simulink model "Week11_Simulation_Control"  (R2017b)
settings: Solver=ode4  StartTime=0.0  StopTime=20  FixedStep=1e-3  RelTol=1e-3  EnableMultiTasking=on
values from neighbouring files (symbols this model uses):
  g = 9.8    [Parameters.m]
  l1 = 3    [Parameters.m]
  l2 = 2    [Parameters.m]
  m1 = 3    [Parameters.m]
  m2 = 2    [Parameters.m]
undefined symbols (not defined in the file or in its folder): DiscIntNeverNeededParam
libraries: simulink x16, dspinverses x6
(part 1 of 2)
settings Model: Creator=e27269  LastModifiedBy=e27269
settings DataIOCC: LimitDataPoints=on
settings OptimizationCC: LifeSpan=inf
settings DebuggingCC: AllowSymbolicDim=off  SFUnexpectedBacktrackingDiag=warning  SFNoUnconditionalDefaultTransitionDiag=warning  SFExecutionAtInitializationDiag=none
settings ModelReferenceCC: PropagateSignalLabelsOutOfModel=off
settings CodeAppCC: StateflowObjectComments=on
settings GRTTargetCC: TargetLangStandard=C89/C90 (ANSI)
settings ConfigComp: CovMetricSettings=dw  CovHtmlReporting=on  CovSaveCumulativeToWorkspaceVar=on  CovSaveSingleToWorkspaceVar=on  CovExternalEMLEnable=off

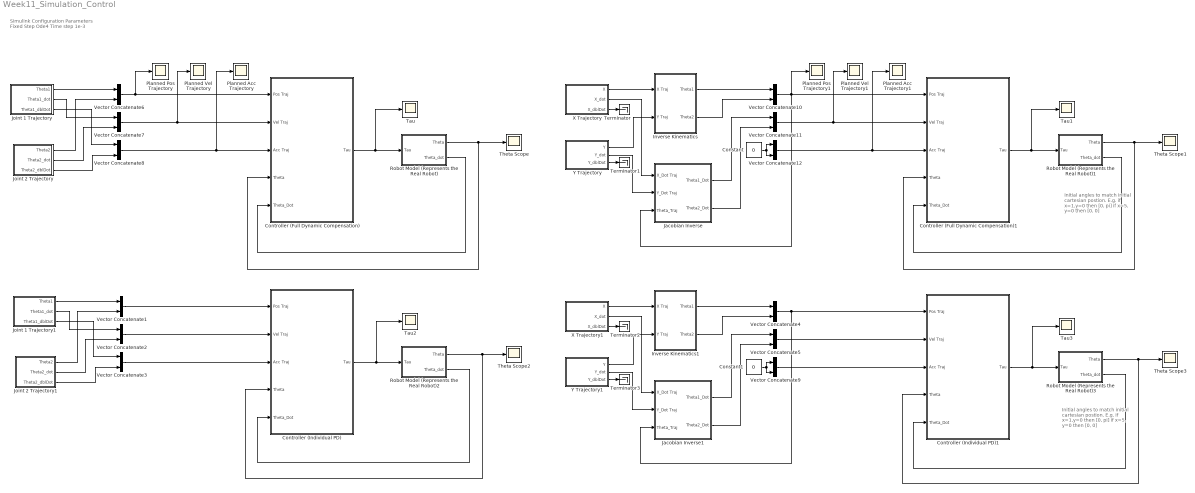
== system Week11_Simulation_Control ==
  note: Simulink Configuration Parameters
      | Fixed Step
      | Ode4
      | Time step 1e-3
  note: Initial angles to
      | match initial
      | cartesian postion.
      | E.g. if x=1,y=0
      | then [0, pi]
      | if x=5, y=0
      | then [0, 0]
  note: Initial angles to
      | match initial
      | cartesian postion.
      | E.g. if x=1,y=0
      | then [0, pi]
      | if x=5, y=0
      | then [0, 0]
  Constant : Constant  Value=0
  Constant1 : Constant  Value=0
  Controller (Full Dynamic Compensation) : Subsystem
  Controller (Full Dynamic Compensation)1 : Subsystem
  Controller (Individual PD) : Subsystem
  Controller (Individual PD)1 : Subsystem
  Inverse Kinematics : Subsystem
  Inverse Kinematics1 : Subsystem
  Jacobian Inverse : Subsystem
  Jacobian Inverse1 : Subsystem
  Joint 1 Trajectory : Subsystem
  Joint 1 Trajectory1 : Subsystem
  Joint 2 Trajectory : Subsystem
  Joint 2 Trajectory1 : Subsystem
  Planned Acc Trajectory : Scope
  Planned Acc Trajectory1 : Scope
  Planned Pos Trajectory : Scope
  Planned Pos Trajectory1 : Scope
  Planned Vel Trajectory : Scope
  Planned Vel Trajectory1 : Scope
  Robot Model (Represents the Real Robot) : Subsystem
  Robot Model (Represents the Real Robot)1 : Subsystem
  Robot Model (Represents the Real Robot)2 : Subsystem
  Robot Model (Represents the Real Robot)3 : Subsystem
  Tau{,1..3} (4 alike) : Scope
  Terminator{,1..3} (4 alike) : Terminator
  Theta Scope{,1..3} (4 alike) : Scope
  Vector Concatenate{1..12} (12 alike) : Concatenate  Mode=Multidimensional array
  X Trajectory : Subsystem
  X Trajectory1 : Subsystem
  Y Trajectory : Subsystem
  Y Trajectory1 : Subsystem
  wires:
  Joint 1 Trajectory/1(Theta1) -> Vector Concatenate6/1
  Joint 2 Trajectory/2(Theta2_dot) -> Vector Concatenate7/2
  Joint 2 Trajectory/1(Theta2) -> Vector Concatenate6/2
  Joint 1 Trajectory/2(Theta1_dot) -> Vector Concatenate7/1
  Joint 1 Trajectory/3(Theta1_dblDot) -> Vector Concatenate8/1
  Joint 2 Trajectory/3(Theta2_dblDot) -> Vector Concatenate8/2
  Vector Concatenate6/1 -> Controller (Full Dynamic Compensation)/1(Pos Traj), Planned Pos Trajectory/1
  Vector Concatenate7/1 -> Planned Vel Trajectory/1, Controller (Full Dynamic Compensation)/2(Vel Traj)
  Robot Model (Represents the Real Robot)/1(Theta) -> Controller (Full Dynamic Compensation)/4(Theta), Theta Scope/1
  Vector Concatenate8/1 -> Planned Acc Trajectory/1, Controller (Full Dynamic Compensation)/3(Acc Traj)
  Controller (Full Dynamic Compensation)/1(Tau) -> Tau/1, Robot Model (Represents the Real Robot)/1(Tau)
  Robot Model (Represents the Real Robot)/2(Theta_dot) -> Controller (Full Dynamic Compensation)/5(Theta_Dot)
  Robot Model (Represents the Real Robot)2/2(Theta_dot) -> Controller (Individual PD)/5(Theta_Dot)
  Controller (Individual PD)/1(Tau) -> Robot Model (Represents the Real Robot)2/1(Tau), Tau2/1
  Robot Model (Represents the Real Robot)2/1(Theta) -> Controller (Individual PD)/4(Theta), Theta Scope2/1
  Joint 2 Trajectory1/3(Theta2_dblDot) -> Vector Concatenate3/2
  Joint 2 Trajectory1/1(Theta2) -> Vector Concatenate1/2
  Joint 1 Trajectory1/3(Theta1_dblDot) -> Vector Concatenate3/1
  Joint 1 Trajectory1/2(Theta1_dot) -> Vector Concatenate2/1
  Joint 2 Trajectory1/2(Theta2_dot) -> Vector Concatenate2/2
  Joint 1 Trajectory1/1(Theta1) -> Vector Concatenate1/1
  Vector Concatenate1/1 -> Controller (Individual PD)/1(Pos Traj)
  Vector Concatenate2/1 -> Controller (Individual PD)/2(Vel Traj)
  Vector Concatenate3/1 -> Controller (Individual PD)/3(Acc Traj)
  Jacobian Inverse1/1(Theta1_Dot) -> Vector Concatenate5/1
  Y Trajectory1/1(Y) -> Inverse Kinematics1/2(Y Traj)
  Inverse Kinematics1/1(Theta1) -> Vector Concatenate4/1
  Vector Concatenate4/1 -> Controller (Individual PD)1/1(Pos Traj), Jacobian Inverse1/3(Theta_Traj)
  Vector Concatenate5/1 -> Controller (Individual PD)1/2(Vel Traj)
  Jacobian Inverse1/2(Theta2_Dot) -> Vector Concatenate5/2
  X Trajectory1/2(X_dot) -> Jacobian Inverse1/1(X_Dot Traj)
  X Trajectory/2(X_dot) -> Jacobian Inverse/1(X_Dot Traj)
  Jacobian Inverse/2(Theta2_Dot) -> Vector Concatenate11/2
  Robot Model (Represents the Real Robot)3/2(Theta_dot) -> Controller (Individual PD)1/5(Theta_Dot)
  Constant/1 -> Vector Concatenate12/2, Vector Concatenate12/1
  Vector Concatenate11/1 -> Planned Vel Trajectory1/1, Controller (Full Dynamic Compensation)1/2(Vel Traj)
  Robot Model (Represents the Real Robot)1/1(Theta) -> Controller (Full Dynamic Compensation)1/4(Theta), Theta Scope1/1
  Vector Concatenate10/1 -> Jacobian Inverse/3(Theta_Traj), Controller (Full Dynamic Compensation)1/1(Pos Traj), Planned Pos Trajectory1/1
  X Trajectory/1(X) -> Inverse Kinematics/1(X Traj)
  Y Trajectory1/3(Y_dblDot) -> Terminator3/1
  Controller (Individual PD)1/1(Tau) -> Robot Model (Represents the Real Robot)3/1(Tau), Tau3/1
  Inverse Kinematics/1(Theta1) -> Vector Concatenate10/1
  Robot Model (Represents the Real Robot)3/1(Theta) -> Controller (Individual PD)1/4(Theta), Theta Scope3/1
  Y Trajectory/1(Y) -> Inverse Kinematics/2(Y Traj)
  Jacobian Inverse/1(Theta1_Dot) -> Vector Concatenate11/1
  Robot Model (Represents the Real Robot)1/2(Theta_dot) -> Controller (Full Dynamic Compensation)1/5(Theta_Dot)
  X Trajectory1/1(X) -> Inverse Kinematics1/1(X Traj)
  Controller (Full Dynamic Compensation)1/1(Tau) -> Tau1/1, Robot Model (Represents the Real Robot)1/1(Tau)
  Vector Concatenate12/1 -> Planned Acc Trajectory1/1, Controller (Full Dynamic Compensation)1/3(Acc Traj)
  Inverse Kinematics/2(Theta2) -> Vector Concatenate10/2
  X Trajectory/3(X_dblDot) -> Terminator/1
  Y Trajectory1/2(Y_dot) -> Jacobian Inverse1/2(Y_Dot Traj)
  Inverse Kinematics1/2(Theta2) -> Vector Concatenate4/2
  Vector Concatenate9/1 -> Controller (Individual PD)1/3(Acc Traj)
  Y Trajectory/3(Y_dblDot) -> Terminator1/1
  X Trajectory1/3(X_dblDot) -> Terminator2/1
  Y Trajectory/2(Y_dot) -> Jacobian Inverse/2(Y_Dot Traj)
  Constant1/1 -> Vector Concatenate9/2, Vector Concatenate9/1

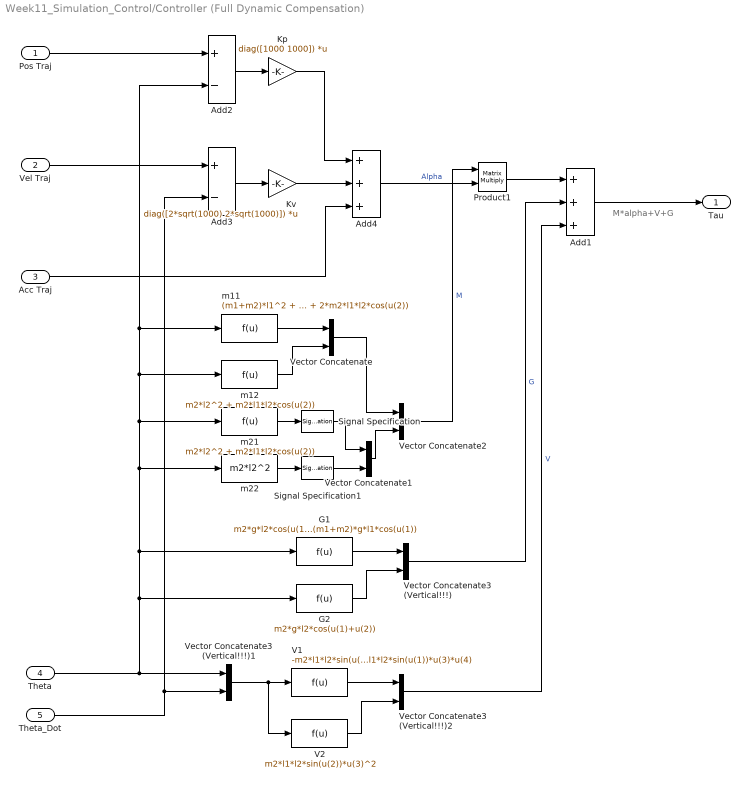
== system Week11_Simulation_Control/Controller (Full Dynamic Compensation) ==
  note: M*alpha+V+G
  Pos Traj : Inport
  Vel Traj : Inport  Port=2
  Acc Traj : Inport  Port=3
  Theta : Inport  Port=4
  Theta_Dot : Inport  Port=5
  Add1 : Sum  Inputs=+++
  Add2 : Sum  Inputs=+-
  Add3 : Sum  Inputs=+-
  Add4 : Sum  Inputs=+++
  G1 : Fcn  Expr=m2*g*l2*cos(u(1)+u(2))+(m1+m2)*g*l1*cos(u(1))
  G2 : Fcn  Expr=m2*g*l2*cos(u(1)+u(2))
  Kp : Gain  Gain=diag([1000 1000])  Multiplication=Matrix(K*u) (u vector)
  Kv : Gain  Gain=diag([2*sqrt(1000) 2*sqrt(1000)])  Multiplication=Matrix(K*u) (u vector)
  Product1 : Product  Multiplication=Matrix(*)
  Signal Specification : SignalSpecification  Dimensions=[1,1]
  Signal Specification1 : SignalSpecification  Dimensions=[1,1]
  V1 : Fcn  Expr=-m2*l1*l2*sin(u(2))*u(4)^2-2*m2*l1*l2*sin(u(1))*u(3)*u(4)
  V2 : Fcn  Expr=m2*l1*l2*sin(u(2))*u(3)^2
  Vector Concatenate : Concatenate  Mode=Multidimensional array  ConcatenateDimension=2
  Vector Concatenate1 : Concatenate  Mode=Multidimensional array  ConcatenateDimension=2
  Vector Concatenate2 : Concatenate  Mode=Multidimensional array
  Vector Concatenate3 (Vertical!!!) : Concatenate  Mode=Multidimensional array
  Vector Concatenate3 (Vertical!!!)1 : Concatenate  Mode=Multidimensional array
  Vector Concatenate3 (Vertical!!!)2 : Concatenate  Mode=Multidimensional array
  m11 : Fcn  Expr=(m1+m2)*l1^2 + m2*l2^2 + 2*m2*l1*l2*cos(u(2))
  m12 : Fcn  Expr=m2*l2^2 + m2*l1*l2*cos(u(2))
  m21 : Fcn  Expr=m2*l2^2 + m2*l1*l2*cos(u(2))
  m22 : Fcn  Expr=m2*l2^2
  Tau : Outport
  wires:
  Vector Concatenate3 (Vertical!!!)2/1 -> Add1/3  "V"
  Vector Concatenate3 (Vertical!!!)1/1 -> V2/1, V1/1
  Theta_Dot/1 -> Vector Concatenate3 (Vertical!!!)1/2, Add3/2
  V1/1 -> Vector Concatenate3 (Vertical!!!)2/1
  Pos Traj/1 -> Add2/1
  Theta/1 -> Add2/2, m11/1, m12/1, m21/1, m22/1, G1/1, G2/1, Vector Concatenate3 (Vertical!!!)1/1
  Signal Specification/1 -> Vector Concatenate1/1
  Vel Traj/1 -> Add3/1
  V2/1 -> Vector Concatenate3 (Vertical!!!)2/2
  Vector Concatenate1/1 -> Vector Concatenate2/2
  Vector Concatenate/1 -> Vector Concatenate2/1
  Signal Specification1/1 -> Vector Concatenate1/2
  m12/1 -> Vector Concatenate/2
  G2/1 -> Vector Concatenate3 (Vertical!!!)/2
  G1/1 -> Vector Concatenate3 (Vertical!!!)/1
  Vector Concatenate2/1 -> Product1/1  "M"
  Acc Traj/1 -> Add4/3
  m22/1 -> Signal Specification1/1
  m11/1 -> Vector Concatenate/1
  m21/1 -> Signal Specification/1
  Add1/1 -> Tau/1
  Vector Concatenate3 (Vertical!!!)/1 -> Add1/2  "G"
  Product1/1 -> Add1/1
  Add2/1 -> Kp/1
  Add3/1 -> Kv/1
  Kv/1 -> Add4/2
  Kp/1 -> Add4/1
  Add4/1 -> Product1/2  "Alpha"

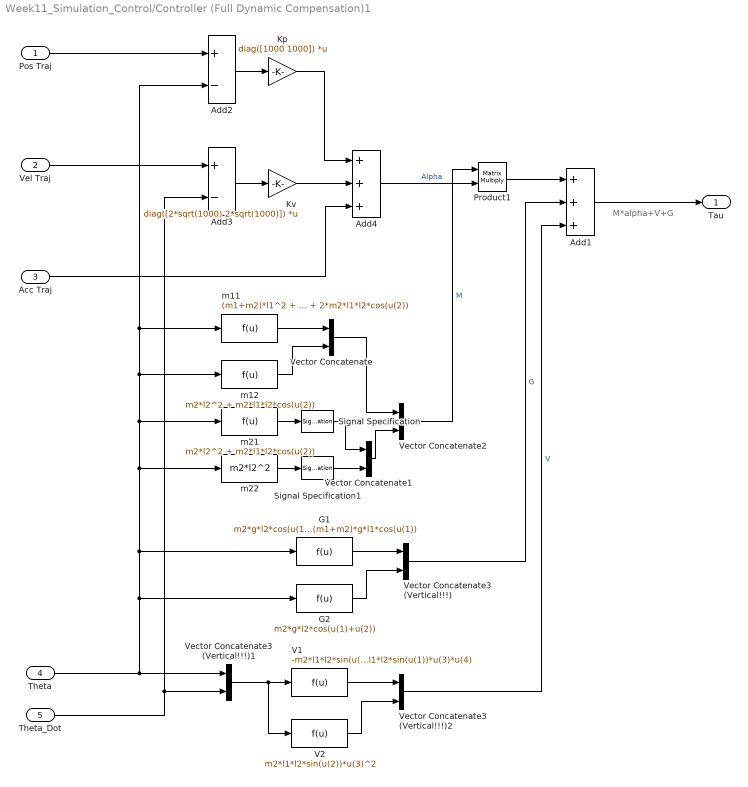
== system Week11_Simulation_Control/Controller (Full Dynamic Compensation)1 ==
  note: M*alpha+V+G
  Pos Traj : Inport
  Vel Traj : Inport  Port=2
  Acc Traj : Inport  Port=3
  Theta : Inport  Port=4
  Theta_Dot : Inport  Port=5
  Add1 : Sum  Inputs=+++
  Add2 : Sum  Inputs=+-
  Add3 : Sum  Inputs=+-
  Add4 : Sum  Inputs=+++
  G1 : Fcn  Expr=m2*g*l2*cos(u(1)+u(2))+(m1+m2)*g*l1*cos(u(1))
  G2 : Fcn  Expr=m2*g*l2*cos(u(1)+u(2))
  Kp : Gain  Gain=diag([1000 1000])  Multiplication=Matrix(K*u) (u vector)
  Kv : Gain  Gain=diag([2*sqrt(1000) 2*sqrt(1000)])  Multiplication=Matrix(K*u) (u vector)
  Product1 : Product  Multiplication=Matrix(*)
  Signal Specification : SignalSpecification  Dimensions=[1,1]
  Signal Specification1 : SignalSpecification  Dimensions=[1,1]
  V1 : Fcn  Expr=-m2*l1*l2*sin(u(2))*u(4)^2-2*m2*l1*l2*sin(u(1))*u(3)*u(4)
  V2 : Fcn  Expr=m2*l1*l2*sin(u(2))*u(3)^2
  Vector Concatenate : Concatenate  Mode=Multidimensional array  ConcatenateDimension=2
  Vector Concatenate1 : Concatenate  Mode=Multidimensional array  ConcatenateDimension=2
  Vector Concatenate2 : Concatenate  Mode=Multidimensional array
  Vector Concatenate3 (Vertical!!!) : Concatenate  Mode=Multidimensional array
  Vector Concatenate3 (Vertical!!!)1 : Concatenate  Mode=Multidimensional array
  Vector Concatenate3 (Vertical!!!)2 : Concatenate  Mode=Multidimensional array
  m11 : Fcn  Expr=(m1+m2)*l1^2 + m2*l2^2 + 2*m2*l1*l2*cos(u(2))
  m12 : Fcn  Expr=m2*l2^2 + m2*l1*l2*cos(u(2))
  m21 : Fcn  Expr=m2*l2^2 + m2*l1*l2*cos(u(2))
  m22 : Fcn  Expr=m2*l2^2
  Tau : Outport
  wires:
  Vector Concatenate3 (Vertical!!!)2/1 -> Add1/3  "V"
  Vector Concatenate3 (Vertical!!!)1/1 -> V2/1, V1/1
  Theta_Dot/1 -> Vector Concatenate3 (Vertical!!!)1/2, Add3/2
  V1/1 -> Vector Concatenate3 (Vertical!!!)2/1
  Pos Traj/1 -> Add2/1
  Theta/1 -> Add2/2, m11/1, m12/1, m21/1, m22/1, G1/1, G2/1, Vector Concatenate3 (Vertical!!!)1/1
  Signal Specification/1 -> Vector Concatenate1/1
  Vel Traj/1 -> Add3/1
  V2/1 -> Vector Concatenate3 (Vertical!!!)2/2
  Vector Concatenate1/1 -> Vector Concatenate2/2
  Vector Concatenate/1 -> Vector Concatenate2/1
  Signal Specification1/1 -> Vector Concatenate1/2
  m12/1 -> Vector Concatenate/2
  G2/1 -> Vector Concatenate3 (Vertical!!!)/2
  G1/1 -> Vector Concatenate3 (Vertical!!!)/1
  Vector Concatenate2/1 -> Product1/1  "M"
  Acc Traj/1 -> Add4/3
  m22/1 -> Signal Specification1/1
  m11/1 -> Vector Concatenate/1
  m21/1 -> Signal Specification/1
  Add1/1 -> Tau/1
  Vector Concatenate3 (Vertical!!!)/1 -> Add1/2  "G"
  Product1/1 -> Add1/1
  Add2/1 -> Kp/1
  Add3/1 -> Kv/1
  Kv/1 -> Add4/2
  Kp/1 -> Add4/1
  Add4/1 -> Product1/2  "Alpha"

== system Week11_Simulation_Control/Controller (Individual PD) ==
  Pos Traj : Inport
  Vel Traj : Inport  Port=2
  Acc Traj : Inport  Port=3
  Theta : Inport  Port=4
  Theta_Dot : Inport  Port=5
  Add2 : Sum  Inputs=+-
  Add3 : Sum  Inputs=+-
  Add4 : Sum  Inputs=+++
  Kp : Gain  Gain=diag([4000 4000])  Multiplication=Matrix(K*u) (u vector)
  Kv : Gain  Gain=diag([2*sqrt(4000) 2*sqrt(4000)])  Multiplication=Matrix(K*u) (u vector)
  Tau : Outport
  wires:
  Theta_Dot/1 -> Add3/2
  Pos Traj/1 -> Add2/1
  Theta/1 -> Add2/2
  Vel Traj/1 -> Add3/1
  Acc Traj/1 -> Add4/3
  Add2/1 -> Kp/1
  Add3/1 -> Kv/1
  Kv/1 -> Add4/2
  Kp/1 -> Add4/1
  Add4/1 -> Tau/1  "PD Control"

== system Week11_Simulation_Control/Controller (Individual PD)1 ==
  Pos Traj : Inport
  Vel Traj : Inport  Port=2
  Acc Traj : Inport  Port=3
  Theta : Inport  Port=4
  Theta_Dot : Inport  Port=5
  Add2 : Sum  Inputs=+-
  Add3 : Sum  Inputs=+-
  Add4 : Sum  Inputs=+++
  Kp : Gain  Gain=diag([4000 4000])  Multiplication=Matrix(K*u) (u vector)
  Kv : Gain  Gain=diag([2*sqrt(4000) 2*sqrt(4000)])  Multiplication=Matrix(K*u) (u vector)
  Tau : Outport
  wires:
  Theta_Dot/1 -> Add3/2
  Pos Traj/1 -> Add2/1
  Theta/1 -> Add2/2
  Vel Traj/1 -> Add3/1
  Acc Traj/1 -> Add4/3
  Add2/1 -> Kp/1
  Add3/1 -> Kv/1
  Kv/1 -> Add4/2
  Kp/1 -> Add4/1
  Add4/1 -> Tau/1  "PD Control"

== system Week11_Simulation_Control/Inverse Kinematics ==
  X Traj : Inport
  Y Traj : Inport  Port=2
  Add : Sum  Inputs=++--
  Add2 : Sum  Inputs=+++-
  Add3 : Sum
  Add4 : Sum  Inputs=+-
  Constant : Constant  Value=l1^2
  Constant1 : Constant  Value=l2^2
  Constant2 : Constant  Value=2*l1*l2
  Constant3 : Constant  Value=l1^2
  Constant4 : Constant  Value=l2^2
  Constant5 : Constant  Value=2*l1
  Divide : Product  Inputs=*/
  Divide1 : Product  Inputs=*//
  Product : Product
  Product1 : Product
  Sqrt : Sqrt  SaturateOnIntegerOverflow=on
  Trigonometric Function : Trigonometry  Operator=acos
  Trigonometric Function1 : Trigonometry  Operator=atan2
  Trigonometric Function2 : Trigonometry  Operator=acos
  Theta1 : Outport
  Theta2 : Outport  Port=2
  wires:
  X Traj/1 -> Trigonometric Function1/2, Product/2, Product/1  "x"
  Y Traj/1 -> Trigonometric Function1/1, Product1/2, Product1/1  "y"
  Product/1 -> Add3/1, Add2/2, Add/1
  Constant/1 -> Add/3
  Constant1/1 -> Add/4
  Add/1 -> Divide/1
  Constant2/1 -> Divide/2
  Divide/1 -> Trigonometric Function/1
  Trigonometric Function/1 -> Theta2/1
  Trigonometric Function1/1 -> Add4/1  "beta"
  Constant3/1 -> Add2/1
  Constant4/1 -> Add2/4
  Add2/1 -> Divide1/1
  Constant5/1 -> Divide1/2
  Product1/1 -> Add3/2, Add2/3, Add/2
  Add3/1 -> Sqrt/1
  Sqrt/1 -> Divide1/3
  Divide1/1 -> Trigonometric Function2/1
  Trigonometric Function2/1 -> Add4/2  "psi"
  Add4/1 -> Theta1/1

== system Week11_Simulation_Control/Inverse Kinematics1 ==
  X Traj : Inport
  Y Traj : Inport  Port=2
  Add : Sum  Inputs=++--
  Add2 : Sum  Inputs=+++-
  Add3 : Sum
  Add4 : Sum  Inputs=+-
  Constant : Constant  Value=l1^2
  Constant1 : Constant  Value=l2^2
  Constant2 : Constant  Value=2*l1*l2
  Constant3 : Constant  Value=l1^2
  Constant4 : Constant  Value=l2^2
  Constant5 : Constant  Value=2*l1
  Divide : Product  Inputs=*/
  Divide1 : Product  Inputs=*//
  Product : Product
  Product1 : Product
  Sqrt : Sqrt  SaturateOnIntegerOverflow=on
  Trigonometric Function : Trigonometry  Operator=acos
  Trigonometric Function1 : Trigonometry  Operator=atan2
  Trigonometric Function2 : Trigonometry  Operator=acos
  Theta1 : Outport
  Theta2 : Outport  Port=2
  wires:
  X Traj/1 -> Trigonometric Function1/2, Product/2, Product/1  "x"
  Y Traj/1 -> Trigonometric Function1/1, Product1/2, Product1/1  "y"
  Product/1 -> Add3/1, Add2/2, Add/1
  Constant/1 -> Add/3
  Constant1/1 -> Add/4
  Add/1 -> Divide/1
  Constant2/1 -> Divide/2
  Divide/1 -> Trigonometric Function/1
  Trigonometric Function/1 -> Theta2/1
  Trigonometric Function1/1 -> Add4/1  "beta"
  Constant3/1 -> Add2/1
  Constant4/1 -> Add2/4
  Add2/1 -> Divide1/1
  Constant5/1 -> Divide1/2
  Product1/1 -> Add3/2, Add2/3, Add/2
  Add3/1 -> Sqrt/1
  Sqrt/1 -> Divide1/3
  Divide1/1 -> Trigonometric Function2/1
  Trigonometric Function2/1 -> Add4/2  "psi"
  Add4/1 -> Theta1/1

== system Week11_Simulation_Control/Jacobian Inverse ==
  note: vertical
  note: vertical
  note: horizontal
  note: horizontal
  X_Dot Traj : Inport
  Y_Dot Traj : Inport  Port=2
  Theta_Traj : Inport  Port=3
  Demux : Demux  Outputs=2
  J11 : Fcn  Expr=-l1*sin(u(1))-l2*sin(u(1)+u(2))
  J12 : Fcn  Expr=-l2*sin(u(1)+u(2))
  J21 : Fcn  Expr=l1*cos(u(1))+l2*cos(u(1)+u(2))
  J22 : Fcn  Expr=l2*cos(u(1)+u(2))
  Product : Product  Multiplication=Matrix(*)
  Pseudoinverse : dspinverses/Pseudoinverse  wanterr=off  SimulateUsing=Interpreted execution
      settings: SourceProductName=DSP System Toolbox  SourceProductBaseCode=DS
  Vector Concatenate : Concatenate  Mode=Multidimensional array  ConcatenateDimension=2
  Vector Concatenate1 : Concatenate  Mode=Multidimensional array  ConcatenateDimension=2
  Vector Concatenate2 : Concatenate  Mode=Multidimensional array
  Vector Concatenate3 : Concatenate  Mode=Multidimensional array
  Theta1_Dot : Outport
  Theta2_Dot : Outport  Port=2
  wires:
  Theta_Traj/1 -> J21/1, J22/1, J12/1, J11/1
  J11/1 -> Vector Concatenate/1
  J12/1 -> Vector Concatenate/2
  J21/1 -> Vector Concatenate1/1
  J22/1 -> Vector Concatenate1/2
  Vector Concatenate/1 -> Vector Concatenate2/1
  Vector Concatenate1/1 -> Vector Concatenate2/2
  Vector Concatenate2/1 -> Pseudoinverse/1  "J"
  X_Dot Traj/1 -> Vector Concatenate3/1  "x_dot"
  Y_Dot Traj/1 -> Vector Concatenate3/2  "y_dot"
  Pseudoinverse/1 -> Product/1  "Jinv"
  Vector Concatenate3/1 -> Product/2  "v"
  Product/1 -> Demux/1
  Demux/1 -> Theta1_Dot/1
  Demux/2 -> Theta2_Dot/1

== system Week11_Simulation_Control/Jacobian Inverse1 ==
  note: vertical
  note: vertical
  note: horizontal
  note: horizontal
  X_Dot Traj : Inport
  Y_Dot Traj : Inport  Port=2
  Theta_Traj : Inport  Port=3
  Demux : Demux  Outputs=2
  J11 : Fcn  Expr=-l1*sin(u(1))-l2*sin(u(1)+u(2))
  J12 : Fcn  Expr=-l2*sin(u(1)+u(2))
  J21 : Fcn  Expr=l1*cos(u(1))+l2*cos(u(1)+u(2))
  J22 : Fcn  Expr=l2*cos(u(1)+u(2))
  Product : Product  Multiplication=Matrix(*)
  Pseudoinverse : dspinverses/Pseudoinverse  wanterr=off  SimulateUsing=Interpreted execution
      settings: SourceProductName=DSP System Toolbox  SourceProductBaseCode=DS
  Vector Concatenate : Concatenate  Mode=Multidimensional array  ConcatenateDimension=2
  Vector Concatenate1 : Concatenate  Mode=Multidimensional array  ConcatenateDimension=2
  Vector Concatenate2 : Concatenate  Mode=Multidimensional array
  Vector Concatenate3 : Concatenate  Mode=Multidimensional array
  Theta1_Dot : Outport
  Theta2_Dot : Outport  Port=2
  wires:
  Theta_Traj/1 -> J21/1, J22/1, J12/1, J11/1
  J11/1 -> Vector Concatenate/1
  J12/1 -> Vector Concatenate/2
  J21/1 -> Vector Concatenate1/1
  J22/1 -> Vector Concatenate1/2
  Vector Concatenate/1 -> Vector Concatenate2/1
  Vector Concatenate1/1 -> Vector Concatenate2/2
  Vector Concatenate2/1 -> Pseudoinverse/1  "J"
  X_Dot Traj/1 -> Vector Concatenate3/1  "x_dot"
  Y_Dot Traj/1 -> Vector Concatenate3/2  "y_dot"
  Pseudoinverse/1 -> Product/1  "Jinv"
  Vector Concatenate3/1 -> Product/2  "v"
  Product/1 -> Demux/1
  Demux/1 -> Theta1_Dot/1
  Demux/2 -> Theta2_Dot/1

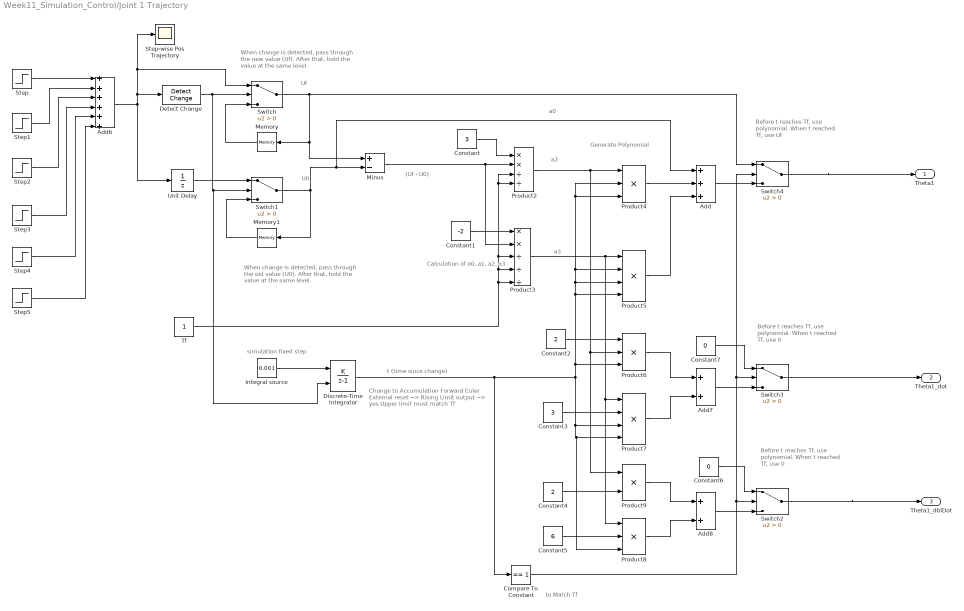
== system Week11_Simulation_Control/Joint 1 Trajectory ==
  note: Generate Polynomial
  note: Calculation of
      | a0, a1, a2, a3
  note: Before t reaches Tf,
      | use polynomial.
      | When t reached Tf,
      | use Uf
  note: to Match Tf
  note: t (time since change)
  note: When change is detected, pass through
      | the old value (U0). After that, hold the
      | value at the same level.
  note: simulation fixed step
  note: Change to Accumulation Forward Euler
      | External reset --> Rising
      | Limit output --> yes
      | Upper limit must match Tf
  note: a3
  note: a2
  note: Uf
  note: U0
  note: When change is detected, pass through
      | the new value (Uf). After that, hold the
      | value at the same level.
  note: Before t reaches Tf,
      | use polynomial.
      | When t reached Tf,
      | use 0
  note: Before t reaches Tf,
      | use polynomial.
      | When t reached Tf,
      | use 0
  note: (Uf - U0)
  note: a0
  Add : Sum  Inputs=3
  Add6 : Sum  Inputs=6
  Add7 : Sum  Inputs=2
  Add8 : Sum  Inputs=2
  Compare To Constant : simulink/Logic and Bit Operations/Compare To Constant  relop===  const=1  OutDataTypeStr=boolean
  Constant : Constant  Value=3
  Constant1 : Constant  Value=-2
  Constant2 : Constant  Value=2
  Constant3 : Constant  Value=3
  Constant4 : Constant  Value=2
  Constant5 : Constant  Value=6
  Constant6 : Constant  Value=0
  Constant7 : Constant  Value=0
  Detect Change : simulink/Logic and Bit Operations/Detect Change  vinit=0  InputProcessing=Inherited  OutDataTypeStr=boolean
  Discrete-Time Integrator : DiscreteIntegrator  IntegratorMethod=Accumulation: Forward Euler  gainval=1  ExternalReset=rising  InitialConditionSetting=State (most efficient)  SampleTime=-1  LimitOutput=on  UpperSaturationLimit=1  ICPrevOutput=DiscIntNeverNeededParam  ICPrevScaledInput=DiscIntNeverNeededParam
  Integral source : Constant  Value=0.001
  Memory : Memory  InheritSampleTime=on
  Memory1 : Memory  InheritSampleTime=on
  Minus : Sum  Inputs=+-
  Product2 : Product  Inputs=**//
  Product3 : Product  Inputs=**///
  Product4 : Product  Inputs=3
  Product5 : Product  Inputs=4
  Product6 : Product  Inputs=3
  Product7 : Product  Inputs=4
  Product8 : Product  Inputs=3
  Product9 : Product
  Step : Step  SampleTime=0
  Step-wise Pos Trajectory : Scope
  Step1 : Step  Time=4  After=2  SampleTime=0
  Step2 : Step  Time=8  After=-1  SampleTime=0
  Step3 : Step  Time=11  After=1.5  SampleTime=0
  Step4 : Step  Time=14  After=-1  SampleTime=0
  Step5 : Step  Time=17  After=-2  SampleTime=0
  Switch{,1..4} (5 alike) : Switch  Criteria=u2 > Threshold
  Tf : Constant
  Unit Delay : UnitDelay  SampleTime=-1
  Theta1 : Outport
  Theta1_dot : Outport  Port=2
  Theta1_dblDot : Outport  Port=3
  wires:
  Add8/1 -> Switch2/3
  Product9/1 -> Add8/1
  Constant7/1 -> Switch3/1
  Constant/1 -> Product2/1
  Step/1 -> Add6/1
  Integral source/1 -> Discrete-Time Integrator/1
  Switch4/1 -> Theta1/1
  Add/1 -> Switch4/3
  Add6/1 -> Switch/1, Step-wise Pos Trajectory/1, Detect Change/1, Unit Delay/1
  Product4/1 -> Add/2
  Switch3/1 -> Theta1_dot/1
  Compare To Constant/1 -> Switch4/2, Switch3/2, Switch2/2
  Switch2/1 -> Theta1_dblDot/1
  Step5/1 -> Add6/6
  Constant6/1 -> Switch2/1
  Step3/1 -> Add6/4
  Constant4/1 -> Product9/2
  Product8/1 -> Add8/2
  Constant5/1 -> Product8/2
  Product5/1 -> Add/3
  Product7/1 -> Add7/2
  Constant3/1 -> Product7/2
  Step4/1 -> Add6/5
  Detect Change/1 -> Discrete-Time Integrator/2, Switch1/2, Switch/2
  Step1/1 -> Add6/2
  Discrete-Time Integrator/1 -> Compare To Constant/1, Product7/3, Product8/3, Product7/4, Product6/3, Product5/4, Product5/3, Product5/2, Product4/3, Product4/2
  Product3/1 -> Product8/1, Product7/1, Product5/1
  Constant1/1 -> Product3/1
  Product6/1 -> Add7/1
  Tf/1 -> Product3/5, Product3/4, Product3/3, Product2/4, Product2/3
  Add7/1 -> Switch3/3
  Step2/1 -> Add6/3
  Minus/1 -> Product3/2, Product2/2
  Unit Delay/1 -> Switch1/1
  Memory1/1 -> Switch1/3
  Switch1/1 -> Memory1/1, Add/1, Minus/2
  Constant2/1 -> Product6/1
  Product2/1 -> Product9/1, Product6/2, Product4/1
  Memory/1 -> Switch/3
  Switch/1 -> Minus/1, Memory/1, Switch4/1

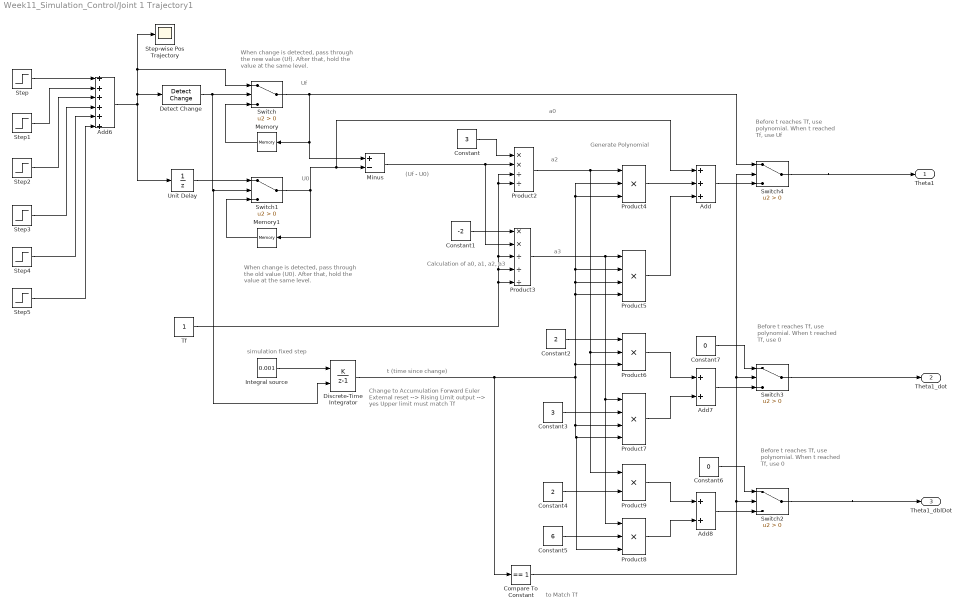
== system Week11_Simulation_Control/Joint 1 Trajectory1 ==
  note: Generate Polynomial
  note: Calculation of
      | a0, a1, a2, a3
  note: Before t reaches Tf,
      | use polynomial.
      | When t reached Tf,
      | use Uf
  note: to Match Tf
  note: t (time since change)
  note: When change is detected, pass through
      | the old value (U0). After that, hold the
      | value at the same level.
  note: simulation fixed step
  note: Change to Accumulation Forward Euler
      | External reset --> Rising
      | Limit output --> yes
      | Upper limit must match Tf
  note: a3
  note: a2
  note: Uf
  note: U0
  note: When change is detected, pass through
      | the new value (Uf). After that, hold the
      | value at the same level.
  note: Before t reaches Tf,
      | use polynomial.
      | When t reached Tf,
      | use 0
  note: Before t reaches Tf,
      | use polynomial.
      | When t reached Tf,
      | use 0
  note: (Uf - U0)
  note: a0
  Add : Sum  Inputs=3
  Add6 : Sum  Inputs=6
  Add7 : Sum  Inputs=2
  Add8 : Sum  Inputs=2
  Compare To Constant : simulink/Logic and Bit Operations/Compare To Constant  relop===  const=1  OutDataTypeStr=boolean
  Constant : Constant  Value=3
  Constant1 : Constant  Value=-2
  Constant2 : Constant  Value=2
  Constant3 : Constant  Value=3
  Constant4 : Constant  Value=2
  Constant5 : Constant  Value=6
  Constant6 : Constant  Value=0
  Constant7 : Constant  Value=0
  Detect Change : simulink/Logic and Bit Operations/Detect Change  vinit=0  InputProcessing=Inherited  OutDataTypeStr=boolean
  Discrete-Time Integrator : DiscreteIntegrator  IntegratorMethod=Accumulation: Forward Euler  gainval=1  ExternalReset=rising  InitialConditionSetting=State (most efficient)  SampleTime=-1  LimitOutput=on  UpperSaturationLimit=1  ICPrevOutput=DiscIntNeverNeededParam  ICPrevScaledInput=DiscIntNeverNeededParam
  Integral source : Constant  Value=0.001
  Memory : Memory  InheritSampleTime=on
  Memory1 : Memory  InheritSampleTime=on
  Minus : Sum  Inputs=+-
  Product2 : Product  Inputs=**//
  Product3 : Product  Inputs=**///
  Product4 : Product  Inputs=3
  Product5 : Product  Inputs=4
  Product6 : Product  Inputs=3
  Product7 : Product  Inputs=4
  Product8 : Product  Inputs=3
  Product9 : Product
  Step : Step  SampleTime=0
  Step-wise Pos Trajectory : Scope
  Step1 : Step  Time=4  After=2  SampleTime=0
  Step2 : Step  Time=8  After=-1  SampleTime=0
  Step3 : Step  Time=11  After=1.5  SampleTime=0
  Step4 : Step  Time=14  After=-1  SampleTime=0
  Step5 : Step  Time=17  After=-2  SampleTime=0
  Switch{,1..4} (5 alike) : Switch  Criteria=u2 > Threshold
  Tf : Constant
  Unit Delay : UnitDelay  SampleTime=-1
  Theta1 : Outport
  Theta1_dot : Outport  Port=2
  Theta1_dblDot : Outport  Port=3
  wires:
  Add8/1 -> Switch2/3
  Product9/1 -> Add8/1
  Constant7/1 -> Switch3/1
  Constant/1 -> Product2/1
  Step/1 -> Add6/1
  Integral source/1 -> Discrete-Time Integrator/1
  Switch4/1 -> Theta1/1
  Add/1 -> Switch4/3
  Add6/1 -> Switch/1, Step-wise Pos Trajectory/1, Detect Change/1, Unit Delay/1
  Product4/1 -> Add/2
  Switch3/1 -> Theta1_dot/1
  Compare To Constant/1 -> Switch4/2, Switch3/2, Switch2/2
  Switch2/1 -> Theta1_dblDot/1
  Step5/1 -> Add6/6
  Constant6/1 -> Switch2/1
  Step3/1 -> Add6/4
  Constant4/1 -> Product9/2
  Product8/1 -> Add8/2
  Constant5/1 -> Product8/2
  Product5/1 -> Add/3
  Product7/1 -> Add7/2
  Constant3/1 -> Product7/2
  Step4/1 -> Add6/5
  Detect Change/1 -> Discrete-Time Integrator/2, Switch1/2, Switch/2
  Step1/1 -> Add6/2
  Discrete-Time Integrator/1 -> Compare To Constant/1, Product7/3, Product8/3, Product7/4, Product6/3, Product5/4, Product5/3, Product5/2, Product4/3, Product4/2
  Product3/1 -> Product8/1, Product7/1, Product5/1
  Constant1/1 -> Product3/1
  Product6/1 -> Add7/1
  Tf/1 -> Product3/5, Product3/4, Product3/3, Product2/4, Product2/3
  Add7/1 -> Switch3/3
  Step2/1 -> Add6/3
  Minus/1 -> Product3/2, Product2/2
  Unit Delay/1 -> Switch1/1
  Memory1/1 -> Switch1/3
  Switch1/1 -> Memory1/1, Add/1, Minus/2
  Constant2/1 -> Product6/1
  Product2/1 -> Product9/1, Product6/2, Product4/1
  Memory/1 -> Switch/3
  Switch/1 -> Minus/1, Memory/1, Switch4/1

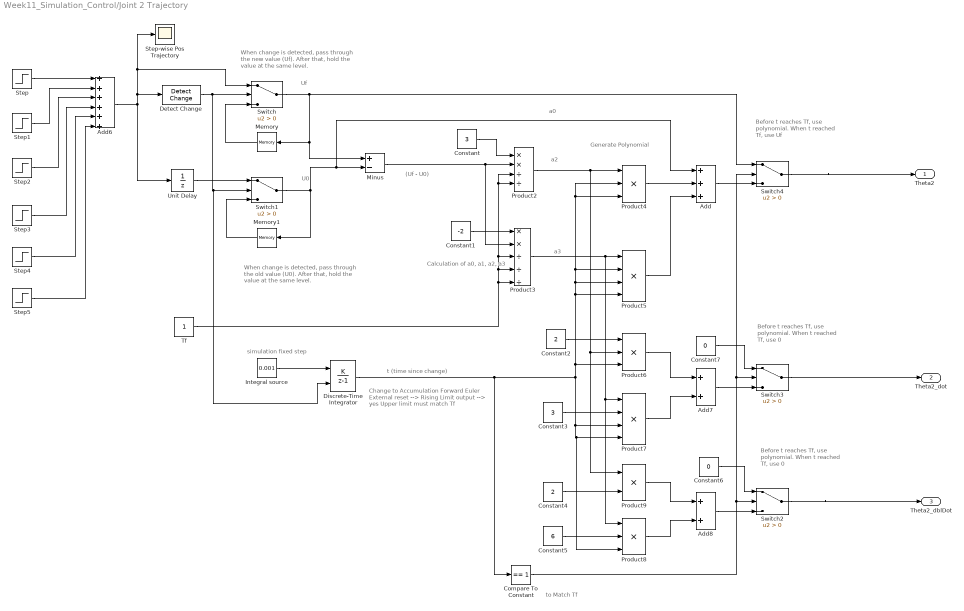
== system Week11_Simulation_Control/Joint 2 Trajectory ==
  note: a0
  note: (Uf - U0)
  note: Before t reaches Tf,
      | use polynomial.
      | When t reached Tf,
      | use 0
  note: Before t reaches Tf,
      | use polynomial.
      | When t reached Tf,
      | use 0
  note: When change is detected, pass through
      | the new value (Uf). After that, hold the
      | value at the same level.
  note: U0
  note: Uf
  note: a2
  note: a3
  note: Change to Accumulation Forward Euler
      | External reset --> Rising
      | Limit output --> yes
      | Upper limit must match Tf
  note: simulation fixed step
  note: When change is detected, pass through
      | the old value (U0). After that, hold the
      | value at the same level.
  note: t (time since change)
  note: to Match Tf
  note: Before t reaches Tf,
      | use polynomial.
      | When t reached Tf,
      | use Uf
  note: Calculation of
      | a0, a1, a2, a3
  note: Generate Polynomial
  Add : Sum  Inputs=3
  Add6 : Sum  Inputs=6
  Add7 : Sum  Inputs=2
  Add8 : Sum  Inputs=2
  Compare To Constant : simulink/Logic and Bit Operations/Compare To Constant  relop===  const=1  OutDataTypeStr=boolean
  Constant : Constant  Value=3
  Constant1 : Constant  Value=-2
  Constant2 : Constant  Value=2
  Constant3 : Constant  Value=3
  Constant4 : Constant  Value=2
  Constant5 : Constant  Value=6
  Constant6 : Constant  Value=0
  Constant7 : Constant  Value=0
  Detect Change : simulink/Logic and Bit Operations/Detect Change  vinit=0  InputProcessing=Inherited  OutDataTypeStr=boolean
  Discrete-Time Integrator : DiscreteIntegrator  IntegratorMethod=Accumulation: Forward Euler  gainval=1  ExternalReset=rising  InitialConditionSetting=State (most efficient)  SampleTime=-1  LimitOutput=on  UpperSaturationLimit=1  ICPrevOutput=DiscIntNeverNeededParam  ICPrevScaledInput=DiscIntNeverNeededParam
  Integral source : Constant  Value=0.001
  Memory : Memory  InheritSampleTime=on
  Memory1 : Memory  InheritSampleTime=on
  Minus : Sum  Inputs=+-
  Product2 : Product  Inputs=**//
  Product3 : Product  Inputs=**///
  Product4 : Product  Inputs=3
  Product5 : Product  Inputs=4
  Product6 : Product  Inputs=3
  Product7 : Product  Inputs=4
  Product8 : Product  Inputs=3
  Product9 : Product
  Step : Step  After=0.5  SampleTime=0
  Step-wise Pos Trajectory : Scope
  Step1 : Step  Time=4  After=1.5  SampleTime=0
  Step2 : Step  Time=8  After=-1  SampleTime=0
  Step3 : Step  Time=12  After=2.5  SampleTime=0
  Step4 : Step  Time=16  After=0.5  SampleTime=0
  Step5 : Step  Time=18  After=-2  SampleTime=0
  Switch{,1..4} (5 alike) : Switch  Criteria=u2 > Threshold
  Tf : Constant
  Unit Delay : UnitDelay  SampleTime=-1
  Theta2 : Outport
  Theta2_dot : Outport  Port=2
  Theta2_dblDot : Outport  Port=3
  wires:
  Switch/1 -> Switch4/1, Memory/1, Minus/1
  Memory/1 -> Switch/3
  Product2/1 -> Product4/1, Product6/2, Product9/1
  Constant2/1 -> Product6/1
  Switch1/1 -> Minus/2, Add/1, Memory1/1
  Memory1/1 -> Switch1/3
  Unit Delay/1 -> Switch1/1
  Minus/1 -> Product2/2, Product3/2
  Step2/1 -> Add6/3
  Add7/1 -> Switch3/3
  Tf/1 -> Product2/3, Product2/4, Product3/3, Product3/4, Product3/5
  Product6/1 -> Add7/1
  Constant1/1 -> Product3/1
  Product3/1 -> Product5/1, Product7/1, Product8/1
  Discrete-Time Integrator/1 -> Product4/2, Product4/3, Product5/2, Product5/3, Product5/4, Product6/3, Product7/4, Product8/3, Product7/3, Compare To Constant/1
  Step1/1 -> Add6/2
  Detect Change/1 -> Switch/2, Switch1/2, Discrete-Time Integrator/2
  Step4/1 -> Add6/5
  Constant3/1 -> Product7/2
  Product7/1 -> Add7/2
  Product5/1 -> Add/3
  Constant5/1 -> Product8/2
  Product8/1 -> Add8/2
  Constant4/1 -> Product9/2
  Step3/1 -> Add6/4
  Constant6/1 -> Switch2/1
  Step5/1 -> Add6/6
  Switch2/1 -> Theta2_dblDot/1
  Compare To Constant/1 -> Switch2/2, Switch3/2, Switch4/2
  Switch3/1 -> Theta2_dot/1
  Product4/1 -> Add/2
  Add6/1 -> Unit Delay/1, Detect Change/1, Step-wise Pos Trajectory/1, Switch/1
  Add/1 -> Switch4/3
  Switch4/1 -> Theta2/1
  Integral source/1 -> Discrete-Time Integrator/1
  Step/1 -> Add6/1
  Constant/1 -> Product2/1
  Constant7/1 -> Switch3/1
  Product9/1 -> Add8/1
  Add8/1 -> Switch2/3

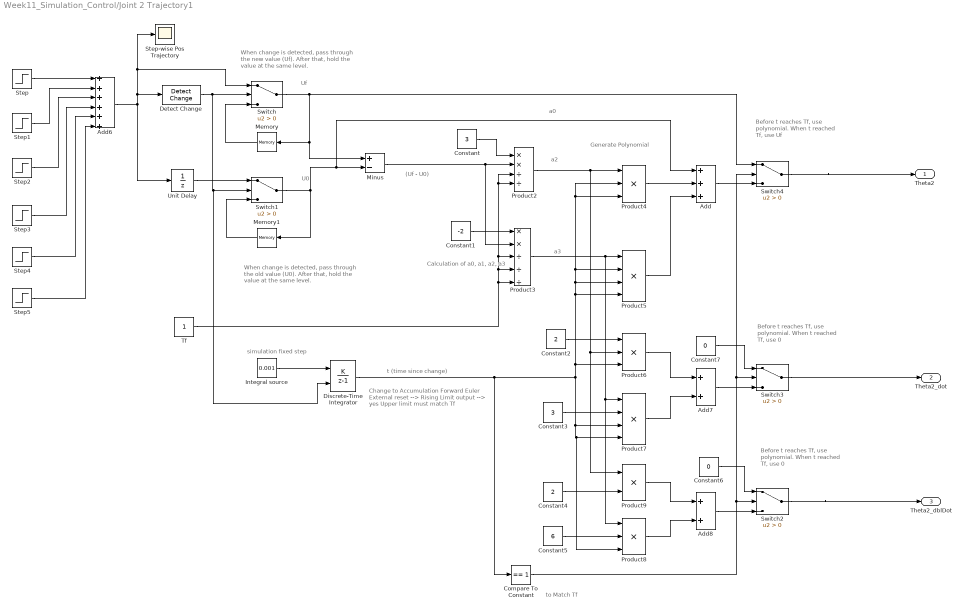
== system Week11_Simulation_Control/Joint 2 Trajectory1 ==
  note: a0
  note: (Uf - U0)
  note: Before t reaches Tf,
      | use polynomial.
      | When t reached Tf,
      | use 0
  note: Before t reaches Tf,
      | use polynomial.
      | When t reached Tf,
      | use 0
  note: When change is detected, pass through
      | the new value (Uf). After that, hold the
      | value at the same level.
  note: U0
  note: Uf
  note: a2
  note: a3
  note: Change to Accumulation Forward Euler
      | External reset --> Rising
      | Limit output --> yes
      | Upper limit must match Tf
  note: simulation fixed step
  note: When change is detected, pass through
      | the old value (U0). After that, hold the
      | value at the same level.
  note: t (time since change)
  note: to Match Tf
  note: Before t reaches Tf,
      | use polynomial.
      | When t reached Tf,
      | use Uf
  note: Calculation of
      | a0, a1, a2, a3
  note: Generate Polynomial
  Add : Sum  Inputs=3
  Add6 : Sum  Inputs=6
  Add7 : Sum  Inputs=2
  Add8 : Sum  Inputs=2
  Compare To Constant : simulink/Logic and Bit Operations/Compare To Constant  relop===  const=1  OutDataTypeStr=boolean
  Constant : Constant  Value=3
  Constant1 : Constant  Value=-2
  Constant2 : Constant  Value=2
  Constant3 : Constant  Value=3
  Constant4 : Constant  Value=2
  Constant5 : Constant  Value=6
  Constant6 : Constant  Value=0
  Constant7 : Constant  Value=0
  Detect Change : simulink/Logic and Bit Operations/Detect Change  vinit=0  InputProcessing=Inherited  OutDataTypeStr=boolean
  Discrete-Time Integrator : DiscreteIntegrator  IntegratorMethod=Accumulation: Forward Euler  gainval=1  ExternalReset=rising  InitialConditionSetting=State (most efficient)  SampleTime=-1  LimitOutput=on  UpperSaturationLimit=1  ICPrevOutput=DiscIntNeverNeededParam  ICPrevScaledInput=DiscIntNeverNeededParam
  Integral source : Constant  Value=0.001
  Memory : Memory  InheritSampleTime=on
  Memory1 : Memory  InheritSampleTime=on
  Minus : Sum  Inputs=+-
  Product2 : Product  Inputs=**//
  Product3 : Product  Inputs=**///
  Product4 : Product  Inputs=3
  Product5 : Product  Inputs=4
  Product6 : Product  Inputs=3
  Product7 : Product  Inputs=4
  Product8 : Product  Inputs=3
  Product9 : Product
  Step : Step  After=0.5  SampleTime=0
  Step-wise Pos Trajectory : Scope
  Step1 : Step  Time=4  After=1.5  SampleTime=0
  Step2 : Step  Time=8  After=-1  SampleTime=0
  Step3 : Step  Time=12  After=2.5  SampleTime=0
  Step4 : Step  Time=16  After=0.5  SampleTime=0
  Step5 : Step  Time=18  After=-2  SampleTime=0
  Switch{,1..4} (5 alike) : Switch  Criteria=u2 > Threshold
  Tf : Constant
  Unit Delay : UnitDelay  SampleTime=-1
  Theta2 : Outport
  Theta2_dot : Outport  Port=2
  Theta2_dblDot : Outport  Port=3
  wires:
  Switch/1 -> Switch4/1, Memory/1, Minus/1
  Memory/1 -> Switch/3
  Product2/1 -> Product4/1, Product6/2, Product9/1
  Constant2/1 -> Product6/1
  Switch1/1 -> Minus/2, Add/1, Memory1/1
  Memory1/1 -> Switch1/3
  Unit Delay/1 -> Switch1/1
  Minus/1 -> Product2/2, Product3/2
  Step2/1 -> Add6/3
  Add7/1 -> Switch3/3
  Tf/1 -> Product2/3, Product2/4, Product3/3, Product3/4, Product3/5
  Product6/1 -> Add7/1
  Constant1/1 -> Product3/1
  Product3/1 -> Product5/1, Product7/1, Product8/1
  Discrete-Time Integrator/1 -> Product4/2, Product4/3, Product5/2, Product5/3, Product5/4, Product6/3, Product7/4, Product8/3, Product7/3, Compare To Constant/1
  Step1/1 -> Add6/2
  Detect Change/1 -> Switch/2, Switch1/2, Discrete-Time Integrator/2
  Step4/1 -> Add6/5
  Constant3/1 -> Product7/2
  Product7/1 -> Add7/2
  Product5/1 -> Add/3
  Constant5/1 -> Product8/2
  Product8/1 -> Add8/2
  Constant4/1 -> Product9/2
  Step3/1 -> Add6/4
  Constant6/1 -> Switch2/1
  Step5/1 -> Add6/6
  Switch2/1 -> Theta2_dblDot/1
  Compare To Constant/1 -> Switch2/2, Switch3/2, Switch4/2
  Switch3/1 -> Theta2_dot/1
  Product4/1 -> Add/2
  Add6/1 -> Unit Delay/1, Detect Change/1, Step-wise Pos Trajectory/1, Switch/1
  Add/1 -> Switch4/3
  Switch4/1 -> Theta2/1
  Integral source/1 -> Discrete-Time Integrator/1
  Step/1 -> Add6/1
  Constant/1 -> Product2/1
  Constant7/1 -> Switch3/1
  Product9/1 -> Add8/1
  Add8/1 -> Switch2/3

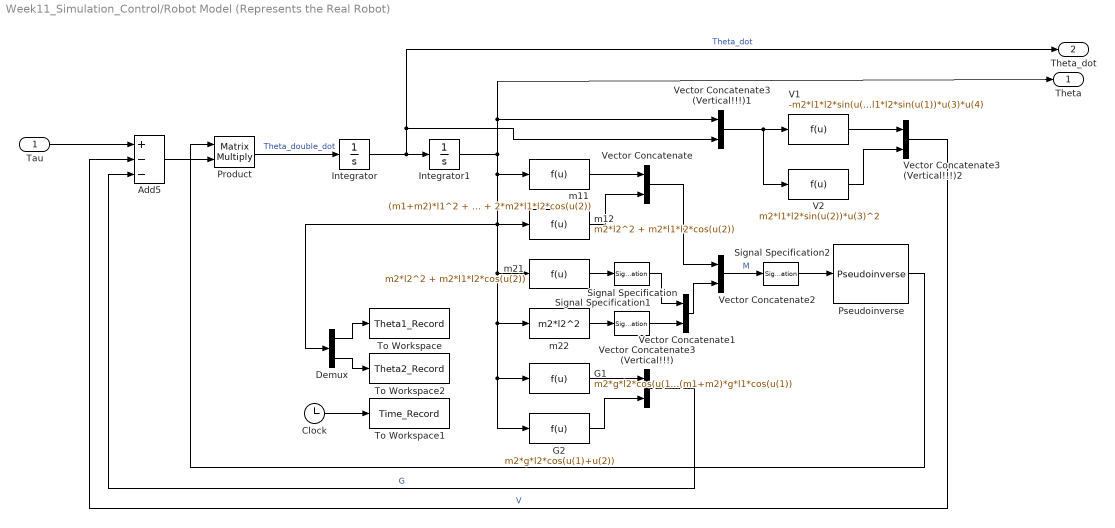
== system Week11_Simulation_Control/Robot Model (Represents the Real Robot) ==
  Tau : Inport
  Add5 : Sum  Inputs=+--
  Clock : Clock
  Demux : Demux  Outputs=2
  G1 : Fcn  Expr=m2*g*l2*cos(u(1)+u(2))+(m1+m2)*g*l1*cos(u(1))
  G2 : Fcn  Expr=m2*g*l2*cos(u(1)+u(2))
  Integrator : Integrator  InitialCondition=[0;0]
  Integrator1 : Integrator  InitialCondition=[0;0.5]
  Product : Product  Multiplication=Matrix(*)
  Pseudoinverse : dspinverses/Pseudoinverse  wanterr=off  SimulateUsing=Interpreted execution
      settings: SourceProductName=DSP System Toolbox  SourceProductBaseCode=DS
  Signal Specification : SignalSpecification  Dimensions=[1,1]
  Signal Specification1 : SignalSpecification  Dimensions=[1,1]
  Signal Specification2 : SignalSpecification  Dimensions=[2,2]
  To Workspace : ToWorkspace  VariableName=Theta1_Record  SampleTime=-1
      settings: Save2DSignal=2-D array (concatenate along first dimension)
  To Workspace1 : ToWorkspace  VariableName=Time_Record  SampleTime=-1
      settings: Save2DSignal=2-D array (concatenate along first dimension)
  To Workspace2 : ToWorkspace  VariableName=Theta2_Record  SampleTime=-1
      settings: Save2DSignal=2-D array (concatenate along first dimension)
  V1 : Fcn  Expr=-m2*l1*l2*sin(u(2))*u(4)^2-2*m2*l1*l2*sin(u(1))*u(3)*u(4)
  V2 : Fcn  Expr=m2*l1*l2*sin(u(2))*u(3)^2
  Vector Concatenate : Concatenate  Mode=Multidimensional array  ConcatenateDimension=2
  Vector Concatenate1 : Concatenate  Mode=Multidimensional array  ConcatenateDimension=2
  Vector Concatenate2 : Concatenate  Mode=Multidimensional array
  Vector Concatenate3 (Vertical!!!) : Concatenate  Mode=Multidimensional array
  Vector Concatenate3 (Vertical!!!)1 : Concatenate  Mode=Multidimensional array
  Vector Concatenate3 (Vertical!!!)2 : Concatenate  Mode=Multidimensional array
  m11 : Fcn  Expr=(m1+m2)*l1^2 + m2*l2^2 + 2*m2*l1*l2*cos(u(2))
  m12 : Fcn  Expr=m2*l2^2 + m2*l1*l2*cos(u(2))
  m21 : Fcn  Expr=m2*l2^2 + m2*l1*l2*cos(u(2))
  m22 : Fcn  Expr=m2*l2^2
  Theta : Outport
  Theta_dot : Outport  Port=2
  wires:
  Tau/1 -> Add5/1
  Integrator/1 -> Theta_dot/1, Vector Concatenate3 (Vertical!!!)1/2, Integrator1/1  "Theta_dot"
  Product/1 -> Integrator/1  "Theta_double_dot"
  Integrator1/1 -> Demux/1, m12/1, m21/1, m22/1, G1/1, G2/1, m11/1, Theta/1, Vector Concatenate3 (Vertical!!!)1/1
  m11/1 -> Vector Concatenate/1
  m12/1 -> Vector Concatenate/2
  m21/1 -> Signal Specification/1
  m22/1 -> Signal Specification1/1
  Vector Concatenate1/1 -> Vector Concatenate2/2
  Vector Concatenate/1 -> Vector Concatenate2/1
  Vector Concatenate2/1 -> Signal Specification2/1  "M"
  G1/1 -> Vector Concatenate3 (Vertical!!!)/1
  G2/1 -> Vector Concatenate3 (Vertical!!!)/2
  Vector Concatenate3 (Vertical!!!)/1 -> Add5/3  "G"
  Vector Concatenate3 (Vertical!!!)1/1 -> V2/1, V1/1
  V1/1 -> Vector Concatenate3 (Vertical!!!)2/1
  V2/1 -> Vector Concatenate3 (Vertical!!!)2/2
  Vector Concatenate3 (Vertical!!!)2/1 -> Add5/2  "V"
  Add5/1 -> Product/2
  Pseudoinverse/1 -> Product/1
  Signal Specification/1 -> Vector Concatenate1/1
  Signal Specification1/1 -> Vector Concatenate1/2
  Signal Specification2/1 -> Pseudoinverse/1
  Clock/1 -> To Workspace1/1
  Demux/1 -> To Workspace/1
  Demux/2 -> To Workspace2/1

== system Week11_Simulation_Control/Robot Model (Represents the Real Robot)1 ==
  note: Set initial
      | angle here
  Tau : Inport
  Add5 : Sum  Inputs=+--
  Demux : Demux  Outputs=2
  G1 : Fcn  Expr=m2*g*l2*cos(u(1)+u(2))+(m1+m2)*g*l1*cos(u(1))
  G2 : Fcn  Expr=m2*g*l2*cos(u(1)+u(2))
  Integrator : Integrator  InitialCondition=[0;0]
  Integrator1 : Integrator  InitialCondition=[0;0]
  Product : Product  Multiplication=Matrix(*)
  Pseudoinverse : dspinverses/Pseudoinverse  wanterr=off  SimulateUsing=Interpreted execution
      settings: SourceProductName=DSP System Toolbox  SourceProductBaseCode=DS
  Signal Specification : SignalSpecification  Dimensions=[1,1]
  Signal Specification1 : SignalSpecification  Dimensions=[1,1]
  Signal Specification2 : SignalSpecification  Dimensions=[2,2]
  To Workspace : ToWorkspace  VariableName=Theta1_RecordC  SampleTime=-1
      settings: Save2DSignal=2-D array (concatenate along first dimension)
  To Workspace2 : ToWorkspace  VariableName=Theta2_RecordC  SampleTime=-1
      settings: Save2DSignal=2-D array (concatenate along first dimension)
  V1 : Fcn  Expr=-m2*l1*l2*sin(u(2))*u(4)^2-2*m2*l1*l2*sin(u(1))*u(3)*u(4)
  V2 : Fcn  Expr=m2*l1*l2*sin(u(2))*u(3)^2
  Vector Concatenate : Concatenate  Mode=Multidimensional array  ConcatenateDimension=2
  Vector Concatenate1 : Concatenate  Mode=Multidimensional array  ConcatenateDimension=2
  Vector Concatenate2 : Concatenate  Mode=Multidimensional array
  Vector Concatenate3 (Vertical!!!) : Concatenate  Mode=Multidimensional array
  Vector Concatenate3 (Vertical!!!)1 : Concatenate  Mode=Multidimensional array
  Vector Concatenate3 (Vertical!!!)2 : Concatenate  Mode=Multidimensional array
  m11 : Fcn  Expr=(m1+m2)*l1^2 + m2*l2^2 + 2*m2*l1*l2*cos(u(2))
  m12 : Fcn  Expr=m2*l2^2 + m2*l1*l2*cos(u(2))
  m21 : Fcn  Expr=m2*l2^2 + m2*l1*l2*cos(u(2))
  m22 : Fcn  Expr=m2*l2^2
  Theta : Outport
  Theta_dot : Outport  Port=2
  wires:
  Tau/1 -> Add5/1
  Integrator/1 -> Theta_dot/1, Vector Concatenate3 (Vertical!!!)1/2, Integrator1/1  "Theta_dot"
  Product/1 -> Integrator/1  "Theta_double_dot"
  Integrator1/1 -> Demux/1, m12/1, m21/1, m22/1, G1/1, G2/1, m11/1, Theta/1, Vector Concatenate3 (Vertical!!!)1/1
  m11/1 -> Vector Concatenate/1
  m12/1 -> Vector Concatenate/2
  m21/1 -> Signal Specification/1
  m22/1 -> Signal Specification1/1
  Vector Concatenate1/1 -> Vector Concatenate2/2
  Vector Concatenate/1 -> Vector Concatenate2/1
  Vector Concatenate2/1 -> Signal Specification2/1  "M"
  G1/1 -> Vector Concatenate3 (Vertical!!!)/1
  G2/1 -> Vector Concatenate3 (Vertical!!!)/2
  Vector Concatenate3 (Vertical!!!)/1 -> Add5/3  "G"
  Vector Concatenate3 (Vertical!!!)1/1 -> V2/1, V1/1
  V1/1 -> Vector Concatenate3 (Vertical!!!)2/1
  V2/1 -> Vector Concatenate3 (Vertical!!!)2/2
  Vector Concatenate3 (Vertical!!!)2/1 -> Add5/2  "V"
  Add5/1 -> Product/2
  Pseudoinverse/1 -> Product/1
  Signal Specification/1 -> Vector Concatenate1/1
  Signal Specification1/1 -> Vector Concatenate1/2
  Signal Specification2/1 -> Pseudoinverse/1
  Demux/1 -> To Workspace/1
  Demux/2 -> To Workspace2/1

== system Week11_Simulation_Control/Robot Model (Represents the Real Robot)2 ==
  Tau : Inport
  Add5 : Sum  Inputs=+--
  Demux : Demux  Outputs=2
  G1 : Fcn  Expr=m2*g*l2*cos(u(1)+u(2))+(m1+m2)*g*l1*cos(u(1))
  G2 : Fcn  Expr=m2*g*l2*cos(u(1)+u(2))
  Integrator : Integrator  InitialCondition=[0;0]
  Integrator1 : Integrator  InitialCondition=[0;0.5]
  Product : Product  Multiplication=Matrix(*)
  Pseudoinverse : dspinverses/Pseudoinverse  wanterr=off  SimulateUsing=Interpreted execution
      settings: SourceProductName=DSP System Toolbox  SourceProductBaseCode=DS
  Signal Specification : SignalSpecification  Dimensions=[1,1]
  Signal Specification1 : SignalSpecification  Dimensions=[1,1]
  Signal Specification2 : SignalSpecification  Dimensions=[2,2]
  To Workspace : ToWorkspace  VariableName=Theta1_RecordB  SampleTime=-1
      settings: Save2DSignal=2-D array (concatenate along first dimension)
  To Workspace2 : ToWorkspace  VariableName=Theta2_RecordB  SampleTime=-1
      settings: Save2DSignal=2-D array (concatenate along first dimension)
  V1 : Fcn  Expr=-m2*l1*l2*sin(u(2))*u(4)^2-2*m2*l1*l2*sin(u(1))*u(3)*u(4)
  V2 : Fcn  Expr=m2*l1*l2*sin(u(2))*u(3)^2
  Vector Concatenate : Concatenate  Mode=Multidimensional array  ConcatenateDimension=2
  Vector Concatenate1 : Concatenate  Mode=Multidimensional array  ConcatenateDimension=2
  Vector Concatenate2 : Concatenate  Mode=Multidimensional array
  Vector Concatenate3 (Vertical!!!) : Concatenate  Mode=Multidimensional array
  Vector Concatenate3 (Vertical!!!)1 : Concatenate  Mode=Multidimensional array
  Vector Concatenate3 (Vertical!!!)2 : Concatenate  Mode=Multidimensional array
  m11 : Fcn  Expr=(m1+m2)*l1^2 + m2*l2^2 + 2*m2*l1*l2*cos(u(2))
  m12 : Fcn  Expr=m2*l2^2 + m2*l1*l2*cos(u(2))
  m21 : Fcn  Expr=m2*l2^2 + m2*l1*l2*cos(u(2))
  m22 : Fcn  Expr=m2*l2^2
  Theta : Outport
  Theta_dot : Outport  Port=2
  wires:
  Tau/1 -> Add5/1
  Integrator/1 -> Theta_dot/1, Vector Concatenate3 (Vertical!!!)1/2, Integrator1/1  "Theta_dot"
  Product/1 -> Integrator/1  "Theta_double_dot"
  Integrator1/1 -> Demux/1, m12/1, m21/1, m22/1, G1/1, G2/1, m11/1, Theta/1, Vector Concatenate3 (Vertical!!!)1/1
  m11/1 -> Vector Concatenate/1
  m12/1 -> Vector Concatenate/2
  m21/1 -> Signal Specification/1
  m22/1 -> Signal Specification1/1
  Vector Concatenate1/1 -> Vector Concatenate2/2
  Vector Concatenate/1 -> Vector Concatenate2/1
  Vector Concatenate2/1 -> Signal Specification2/1  "M"
  G1/1 -> Vector Concatenate3 (Vertical!!!)/1
  G2/1 -> Vector Concatenate3 (Vertical!!!)/2
  Vector Concatenate3 (Vertical!!!)/1 -> Add5/3  "G"
  Vector Concatenate3 (Vertical!!!)1/1 -> V2/1, V1/1
  V1/1 -> Vector Concatenate3 (Vertical!!!)2/1
  V2/1 -> Vector Concatenate3 (Vertical!!!)2/2
  Vector Concatenate3 (Vertical!!!)2/1 -> Add5/2  "V"
  Add5/1 -> Product/2
  Pseudoinverse/1 -> Product/1
  Signal Specification/1 -> Vector Concatenate1/1
  Signal Specification1/1 -> Vector Concatenate1/2
  Signal Specification2/1 -> Pseudoinverse/1
  Demux/1 -> To Workspace/1
  Demux/2 -> To Workspace2/1

== system Week11_Simulation_Control/Robot Model (Represents the Real Robot)3 ==
  note: Set initial
      | angle here
  Tau : Inport
  Add5 : Sum  Inputs=+--
  Demux : Demux  Outputs=2
  G1 : Fcn  Expr=m2*g*l2*cos(u(1)+u(2))+(m1+m2)*g*l1*cos(u(1))
  G2 : Fcn  Expr=m2*g*l2*cos(u(1)+u(2))
  Integrator : Integrator  InitialCondition=[0;0]
  Integrator1 : Integrator  InitialCondition=[0;0]
  Product : Product  Multiplication=Matrix(*)
  Pseudoinverse : dspinverses/Pseudoinverse  wanterr=off  SimulateUsing=Interpreted execution
      settings: SourceProductName=DSP System Toolbox  SourceProductBaseCode=DS
  Signal Specification : SignalSpecification  Dimensions=[1,1]
  Signal Specification1 : SignalSpecification  Dimensions=[1,1]
  Signal Specification2 : SignalSpecification  Dimensions=[2,2]
  To Workspace : ToWorkspace  VariableName=Theta1_RecordD  SampleTime=-1
      settings: Save2DSignal=2-D array (concatenate along first dimension)
  To Workspace2 : ToWorkspace  VariableName=Theta2_RecordD  SampleTime=-1
      settings: Save2DSignal=2-D array (concatenate along first dimension)
  V1 : Fcn  Expr=-m2*l1*l2*sin(u(2))*u(4)^2-2*m2*l1*l2*sin(u(1))*u(3)*u(4)
  V2 : Fcn  Expr=m2*l1*l2*sin(u(2))*u(3)^2
  Vector Concatenate : Concatenate  Mode=Multidimensional array  ConcatenateDimension=2
  Vector Concatenate1 : Concatenate  Mode=Multidimensional array  ConcatenateDimension=2
  Vector Concatenate2 : Concatenate  Mode=Multidimensional array
  Vector Concatenate3 (Vertical!!!) : Concatenate  Mode=Multidimensional array
  Vector Concatenate3 (Vertical!!!)1 : Concatenate  Mode=Multidimensional array
  Vector Concatenate3 (Vertical!!!)2 : Concatenate  Mode=Multidimensional array
  m11 : Fcn  Expr=(m1+m2)*l1^2 + m2*l2^2 + 2*m2*l1*l2*cos(u(2))
  m12 : Fcn  Expr=m2*l2^2 + m2*l1*l2*cos(u(2))
  m21 : Fcn  Expr=m2*l2^2 + m2*l1*l2*cos(u(2))
  m22 : Fcn  Expr=m2*l2^2
  Theta : Outport
  Theta_dot : Outport  Port=2
  wires:
  Tau/1 -> Add5/1
  Integrator/1 -> Theta_dot/1, Vector Concatenate3 (Vertical!!!)1/2, Integrator1/1  "Theta_dot"
  Product/1 -> Integrator/1  "Theta_double_dot"
  Integrator1/1 -> Demux/1, m12/1, m21/1, m22/1, G1/1, G2/1, m11/1, Theta/1, Vector Concatenate3 (Vertical!!!)1/1
  m11/1 -> Vector Concatenate/1
  m12/1 -> Vector Concatenate/2
  m21/1 -> Signal Specification/1
  m22/1 -> Signal Specification1/1
  Vector Concatenate1/1 -> Vector Concatenate2/2
  Vector Concatenate/1 -> Vector Concatenate2/1
  Vector Concatenate2/1 -> Signal Specification2/1  "M"
  G1/1 -> Vector Concatenate3 (Vertical!!!)/1
  G2/1 -> Vector Concatenate3 (Vertical!!!)/2
  Vector Concatenate3 (Vertical!!!)/1 -> Add5/3  "G"
  Vector Concatenate3 (Vertical!!!)1/1 -> V2/1, V1/1
  V1/1 -> Vector Concatenate3 (Vertical!!!)2/1
  V2/1 -> Vector Concatenate3 (Vertical!!!)2/2
  Vector Concatenate3 (Vertical!!!)2/1 -> Add5/2  "V"
  Add5/1 -> Product/2
  Pseudoinverse/1 -> Product/1
  Signal Specification/1 -> Vector Concatenate1/1
  Signal Specification1/1 -> Vector Concatenate1/2
  Signal Specification2/1 -> Pseudoinverse/1
  Demux/1 -> To Workspace/1
  Demux/2 -> To Workspace2/1
